simulink model "actividad_1"  (R2021b)
settings: Solver=VariableStepAuto  StartTime=0.0  StopTime=15  RelTol=1e-3
settings Model: Creator=adana  LastModifiedBy=adana

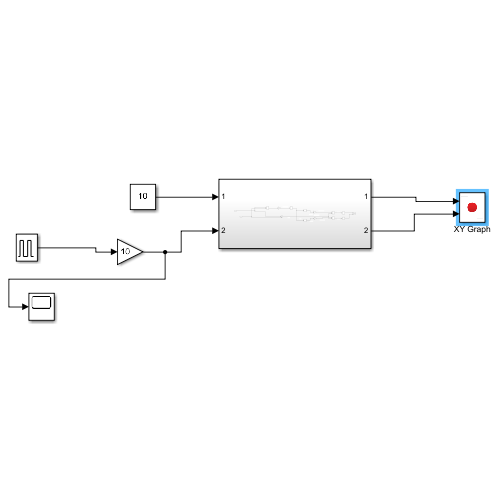
[thumbnail: Simulink's stored preview of the top-level diagram]
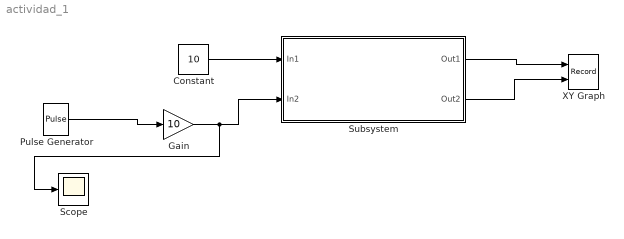
== system actividad_1 ==
  Constant : Constant  Value=10
  Gain : Gain  Gain=10
  Pulse Generator : DiscretePulseGenerator  PulseType=Time based  PulseWidth=80
  Scope : Scope
  Subsystem : Subsystem
  XY Graph : Record  FileSettingsInternal="{\"entries\":[{\"content\":{\"excelSettings\":{\"content\":{},\"type\":\"Streamout.ExcelSettings\"}},\"type\":\"Streamout.FileSettingStorage\",\"uuid\":\"33e0a251-8075-4563-b246-7ef1f729669d\"}],\"packageUris\":[\"http://schema.mathworks.com/mf0/streamout_blocks/R2020a\"],\"version\":\"1.0\"}"  Layout=[1 1]  SignalsInternal="{\"entries\":[{\"content\":{\"signals\":[{\"content\":{\"blockPath\":[\"actividad_1/XY Graph\"],\"channel\":[],\"dimensions\":[1],\"domain\":\"actividad_1/XY Graph\",\"lineColor\":\"#a2142f\",\"plots\":[1],\"port\":1,\"sid\":[\"\"],\"signalID\":1225,\"signalName\":\"Subsystem:1\"},\"type\":\"RecordBlkView.Signal\",\"uuid\":\"a36d2425-c06d-4975-8e9b-d5ed01e0620b\"},{\"content\":{\"blockPath\":[\"actividad_1/XY Graph\"],\"channel\":[],\"dimensions\":[1],\"domain\":\"actividad_1/XY Graph\",\"lineColor\":\"#139fff\",\"plots\":[1],\"port\":2,\"sid\":[\"\"],\"signalID\":1229,\"signalName\":\"Subsystem:2\"},\"type\":\"RecordBlkView.Signal\",\"uuid\":\"4ff6a381-eedb-4dfc-becb-de93018da523\"}]},\"type\":\"RecordBlkView.InputSignals\",\"uuid\":\"ec4ea0f5-1a90-4d0a-8404-42d3bdb0cb09\"}],\"packageUris\":[\"http://schema.mathworks.com/mf0/streamout_blocks/R2020a\"],\"version\":\"1.0\"}"  VisualizationBindings="{\"xyplotplugin\":{\"info\":[{\"series\":[{\"bindingParametersList\":[{\"parameter\":\"X-Axis\",\"signalID\":1225,\"signalName\":\"Subsystem:1\"},{\"parameter\":\"Y-Axis\",\"signalID\":1229,\"signalName\":\"Subsystem:2\"}],\"seriesID\":12040}],\"subplotID\":1}]}}"  CompatibilityTag=XY  st=-1
  wires:
  Constant/1 -> Subsystem/1(In1)
  Subsystem/1(Out1) -> XY Graph/1
  Subsystem/2(Out2) -> XY Graph/2
  Pulse Generator/1 -> Gain/1
  Gain/1 -> Scope/1, Subsystem/2(In2)

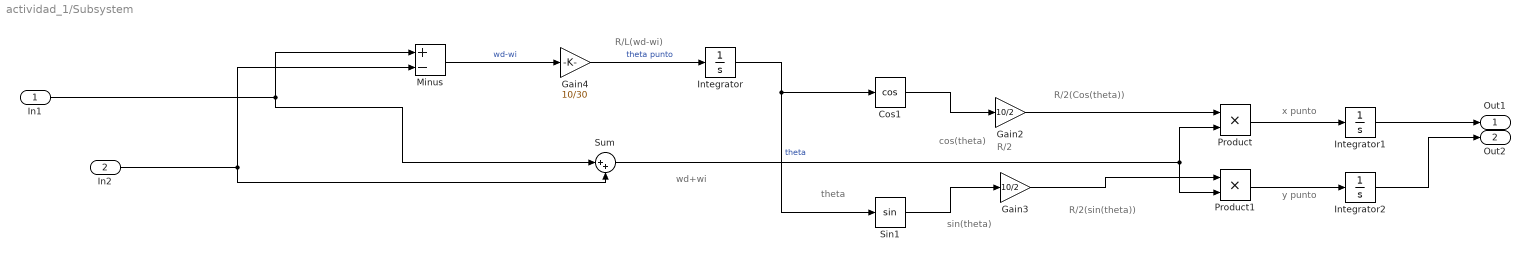
== system actividad_1/Subsystem ==
  note: R/2(sin(theta))
  note: R/2
  note: R/L(wd-wi)
  note: wd+wi
  note: sin(theta)
  note: cos(theta)
  note: R/2(Cos(theta))
  note: x punto
  note: y punto
  note: theta
  In1 : Inport
  In2 : Inport  Port=2
  Cos1 : Trigonometry  Operator=cos
  Gain2 : Gain  Gain=10/2
  Gain3 : Gain  Gain=10/2
  Gain4 : Gain  Gain=10/30
  Integrator : Integrator
  Integrator1 : Integrator
  Integrator2 : Integrator
  Minus : Sum  Inputs=+-
  Product : Product
  Product1 : Product
  Sin1 : Trigonometry
  Sum : Sum  Inputs=|++
  Out1 : Outport
  Out2 : Outport  Port=2
  wires:
  Sum/1 -> Product1/2, Product/2
  Cos1/1 -> Gain2/1
  Product/1 -> Integrator1/1
  Integrator/1 -> Sin1/1, Cos1/1  "theta"
  In1/1 -> Sum/1, Minus/1
  Minus/1 -> Gain4/1  "wd-wi"
  In2/1 -> Sum/2, Minus/2
  Gain4/1 -> Integrator/1  "theta punto"
  Gain2/1 -> Product/1
  Sin1/1 -> Gain3/1
  Gain3/1 -> Product1/1
  Product1/1 -> Integrator2/1
  Integrator2/1 -> Out2/1
  Integrator1/1 -> Out1/1
